simulink model "comp_cic_model"  (R2022b)
settings: Solver=VariableStepAuto  StartTime=0.0  StopTime=2e-3  RelTol=1e-3  EnableMultiTasking=on
values from neighbouring files (symbols this model uses):
  Fcoef = 16    [sim_comp_cic_model.m]
  fo = 5    [sim_comp_cic_model.m]
  fsL = 48    [sim_comp_cic_model.m]
  h_comp_cic = round(h_comp_cic*2^16)*2^-16    [sim_comp_cic_model.m]
  switch_case = 3    [sim_comp_cic_model.m]
  Wcoef = 18    [sim_comp_cic_model.m]
  Win = 16    [sim_comp_cic_model.m]
libraries: dspsrcs4 x2
settings Model: Creator=asperez  LastModifiedBy=smorsua
settings SolverCC: AlgebraicLoopSolver=TrustRegion
settings DataIOCC: ReturnWorkspaceOutputs=off
settings OptimizationCC: LifeSpan=inf
settings DebuggingCC: UnconnectedInputMsg=warning  UnconnectedOutputMsg=warning  UnconnectedLineMsg=warning  SFUnexpectedBacktrackingDiag=warning  SFNoUnconditionalDefaultTransitionDiag=warning  ArithmeticOperatorsInVariantConditions=warning
settings ModelReferenceCC: EnableRefExpFcnMdlSchedulingChecks=on
settings SFSimCC: SimUseLocalCustomCode=off  CustomCodeUndefinedFunction=UseInterfaceOnly
settings RTWCC: RTWUseLocalCustomCode=off
settings CodeAppCC: StateflowObjectComments=on
settings GRTTargetCC: TargetLangStandard=C89/C90 (ANSI)
settings ConfigComp: CovMetricSettings=dw  CovSaveCumulativeToWorkspaceVar=on  CovSaveSingleToWorkspaceVar=on  CovExternalEMLEnable=off

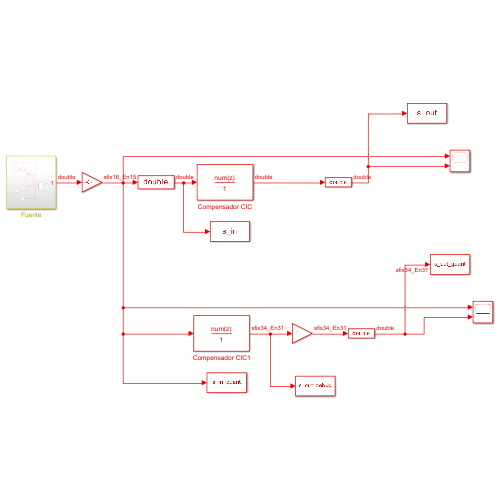
[thumbnail: Simulink's stored preview of the top-level diagram]
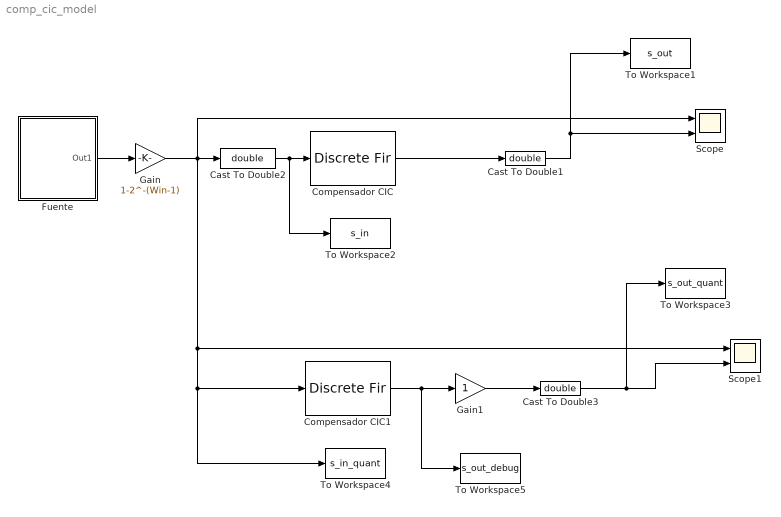
== system comp_cic_model ==
  Cast To Double1 : DataTypeConversion  OutDataTypeStr=double  SaturateOnIntegerOverflow=off  RndMeth=Floor
  Cast To Double2 : DataTypeConversion  OutDataTypeStr=double  SaturateOnIntegerOverflow=off  RndMeth=Floor
  Cast To Double3 : DataTypeConversion  OutDataTypeStr=double  SaturateOnIntegerOverflow=off  RndMeth=Floor
  Compensador CIC : DiscreteFir  Coefficients=h_comp_cic  InputProcessing=Columns as channels (frame based)
  Compensador CIC1 : DiscreteFir  Coefficients=h_comp_cic  InputProcessing=Columns as channels (frame based)  CoefDataTypeStr=fixdt(1,Wcoef,Fcoef)  ProductDataTypeStr=fixdt(1,Wmult,Fmult)  AccumDataTypeStr=fixdt(1,Waccum,Faccum)  OutDataTypeStr=fixdt(1,Wout,Fout)
  Fuente : Subsystem
  Gain : Gain  Gain=1-2^-(Win-1)  ParamDataTypeStr=fixdt(1,16,15)  OutDataTypeStr=fixdt(1,Win,Fin)
  Gain1 : Gain  ParamDataTypeStr=fixdt(1,Wout,Fout)  OutDataTypeStr=fixdt(1,Wout,Fout)
  Scope : Scope  NumInputPorts=2
  Scope1 : Scope  NumInputPorts=2
  To Workspace1 : ToWorkspace  VariableName=s_out  SampleTime=-1
      settings: Save2DSignal=2-D array (concatenate along first dimension)
  To Workspace2 : ToWorkspace  VariableName=s_in  SampleTime=-1
      settings: Save2DSignal=2-D array (concatenate along first dimension)
  To Workspace3 : ToWorkspace  VariableName=s_out_quant  SampleTime=-1
      settings: Save2DSignal=2-D array (concatenate along first dimension)
  To Workspace4 : ToWorkspace  VariableName=s_in_quant  SampleTime=-1
      settings: Save2DSignal=2-D array (concatenate along first dimension)
  To Workspace5 : ToWorkspace  VariableName=s_out_debug  SampleTime=-1
      settings: Save2DSignal=2-D array (concatenate along first dimension)
  wires:
  Fuente/1(Out1) -> Gain/1
  Cast To Double2/1 -> To Workspace2/1, Compensador CIC/1
  Cast To Double1/1 -> Scope/2, To Workspace1/1
  Compensador CIC/1 -> Cast To Double1/1
  Gain/1 -> Scope1/1, Compensador CIC1/1, To Workspace4/1, Scope/1, Cast To Double2/1
  Compensador CIC1/1 -> To Workspace5/1, Gain1/1
  Gain1/1 -> Cast To Double3/1
  Cast To Double3/1 -> To Workspace3/1, Scope1/2

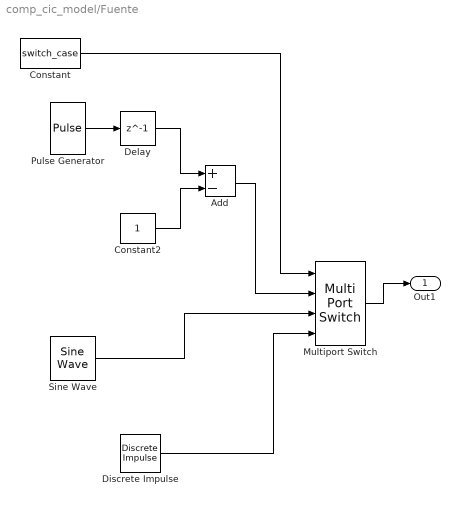
== system comp_cic_model/Fuente ==
  Add : Sum  Inputs=+-
  Constant : Constant  Value=switch_case
  Constant2 : Constant
  Delay : Delay  DelayLength=1  InitialCondition=0  SampleTime=1/(fsL*1000)
  Discrete Impulse : dspsrcs4/Discrete  Impulse  Delay=0  SampleTime=1/(fsL*1000)  FrameSample=1  OutputFrames=off  dataType=double  isSigned=on  wordLen=16  udDataType=sfix(16)  fracBitsMode=Best precision  numFracBits=15  OutDataTypeStr=double  LastOutDataTypeStr=double
  Multiport Switch : MultiPortSwitch  SaturateOnIntegerOverflow=off  InputSameDT=off
  Pulse Generator : DiscretePulseGenerator  PulseType=Time based  Amplitude=2  Period=1/(fo*1000)  PulseWidth=50  SampleTime=1/(fsL*1000)
  Sine Wave : dspsrcs4/Sine Wave  Amplitude=1  Frequency=fo*1000  Phase=0  SampleMode=Discrete  OutComplex=Real  CompMethod=Trigonometric fcn  TableSize=Speed  SampleTime=1/(fsL*1000)  SamplesPerFrame=1  ResetState=Restart at time zero  OutputFrames=on  dataType=double  wordLen=16  udDataType=sfix(16)  fracBitsMode=User-defined  numFracBits=15  OutDataTypeStr=double  LastOutDataTypeStr=double
  Out1 : Outport  VectorParamsAs1DForOutWhenUnconnected=off
  wires:
  Multiport Switch/1 -> Out1/1
  Constant2/1 -> Add/2
  Delay/1 -> Add/1
  Pulse Generator/1 -> Delay/1
  Add/1 -> Multiport Switch/2
  Constant/1 -> Multiport Switch/1
  Discrete Impulse/1 -> Multiport Switch/4
  Sine Wave/1 -> Multiport Switch/3
